simulink model "IdleSpeedSim"  (R2022a)
settings: Solver=FixedStepAuto  StartTime=0.0  StopTime=80  FixedStep=0.01  RelTol=1e-2  EnableMultiTasking=on
InitFcn:
  | IdleSpeedSimParameters
StopFcn:
  | IdleSpeedAutoGrading
values from neighbouring files (symbols this model uses):
  Cd = 0.5    [IdleSpeedSimParameters.m]
  gamma = 1.4    [IdleSpeedSimParameters.m]
  Hu = 42800    [IdleSpeedSimParameters.m]
  J = 1    [IdleSpeedSimParameters.m]
  pambient = 1.013e5    (= 101300)    [IdleSpeedSimParameters.m]
  R = 287e-3    (= 0.287)    [IdleSpeedSimParameters.m]    (also in LQR_Gains.m = [11.13e4 0;0 1])
  T = 294    [IdleSpeedSimParameters.m]
  Vd = 4.6e-3    (= 0.0046)    [IdleSpeedSimParameters.m]
  Vi = 7.36e-3    (= 0.00736)    [IdleSpeedSimParameters.m]
libraries: simulink x1
settings Model: Creator=burl  LastModifiedBy=prajw
settings SolverCC: AlgebraicLoopSolver=TrustRegion
settings DataIOCC: LimitDataPoints=on  SaveFormat=Array  ReturnWorkspaceOutputs=off
settings OptimizationCC: BlockReduction=off  OptimizeBlockIOStorage=off  BufferReuse=off  GlobalBufferReuse=off  ExpressionFolding=off  LocalBlockOutputs=off  LifeSpan=inf  OptimizeDataStoreBuffers=off  BusAssignmentInplaceUpdate=off
settings DebuggingCC: UnderspecifiedInitializationDetection=Classic  MergeDetectMultiDrivingBlocksExec=none  SolverPrmCheckMsg=warning  UnconnectedInputMsg=warning  UnconnectedOutputMsg=warning  UnconnectedLineMsg=warning  StateNameClashWarn=warning  PregeneratedLibrarySubsystemCodeDiagnostic=none  SFUnexpectedBacktrackingDiag=warning  SFNoUnconditionalDefaultTransitionDiag=warning  SFExecutionAtInitializationDiag=none  SFMachineParentedDataDiag=warning  ArithmeticOperatorsInVariantConditions=warning
settings HardwareCC: ProdBitPerPointer=32  ProdBitPerSizeT=32  ProdBitPerPtrDiffT=32  ProdLargestAtomicFloat=None  ProdWordSize=32  ProdHWDeviceType=Generic->Custom  TargetIntDivRoundTo=Zero  TargetEndianess=LittleEndian  TargetHWDeviceType=Generic->Custom
settings ModelReferenceCC: PropagateSignalLabelsOutOfModel=off
settings SFSimCC: SimUseLocalCustomCode=off  CustomCodeUndefinedFunction=UseInterfaceOnly
settings RTWCC: Description=dSPACE DS1006 Hardware Platform  SystemTargetFile=rti1006.tlc  MakeCommand=make_rti  TemplateMakefile=rti1006.tmf  RTWUseLocalCustomCode=off
settings CodeAppCC: StateflowObjectComments=on
settings STFCustomTargetCC: ParMdlRefBuildCompliant=on  MatFileLogging=on  CPPClassGenCompliant=on  SystemTargetFile=rti1006.tlc
settings GRTTargetCC: TargetLangStandard=C89/C90 (ANSI)  CompOptLevelCompliant=off  ConcurrentExecutionCompliant=off  CombineOutputUpdateFcns=off  GRTInterface=on  UseToolchainInfoCompliant=off
settings ConfigComp: CovMetricSettings=dw  CovSaveCumulativeToWorkspaceVar=on  CovSaveSingleToWorkspaceVar=on  CovExternalEMLEnable=off

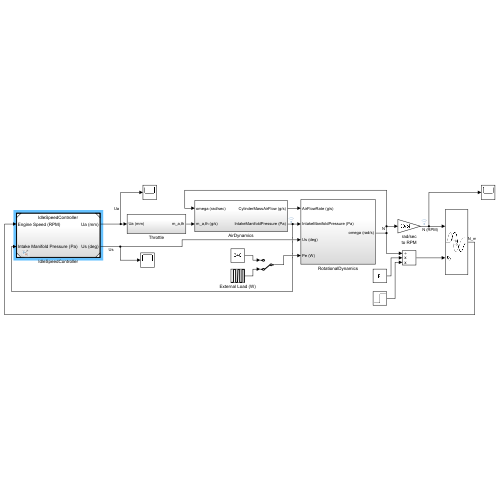
[thumbnail: Simulink's stored preview of the top-level diagram]
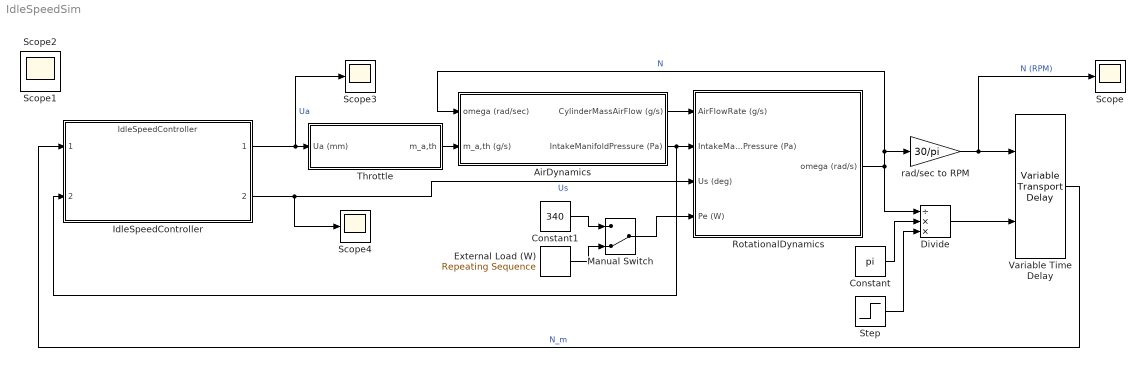
== system IdleSpeedSim ==
  AirDynamics : Subsystem
  Constant : Constant  Value=pi
  Constant1 : Constant  Value=340
  Divide : Product  Inputs=/**
  External Load (W) : simulink/Sources/Repeating Sequence  rep_seq_t=[0 20 20.1 40 40.1]  rep_seq_y=[340 340 1940 1940 340]
  IdleSpeedController : ModelReference  ModelNameDialog=IdleSpeedController  SimulationMode=Normal  ModelReferenceVersion=7.4
  Manual Switch : ManualSwitch  CurrentSetting=0
  RotationalDynamics : Subsystem
  Scope{,1..4} (5 alike) : Scope
  Step : Step  SampleTime=0
  Throttle : Subsystem
  Variable Time Delay : VariableTransportDelay  MaximumDelay=10  ZeroDelay=on
  rad/sec to RPM : Gain  Gain=30/pi
  wires:
  RotationalDynamics/1(omega (rad/s)) -> Divide/1, AirDynamics/1(omega (rad/sec)), rad/sec to RPM/1  "N"
  Variable Time Delay/1 -> IdleSpeedController/1  "N_m"
  IdleSpeedController/1 -> Scope3/1, Throttle/1(Ua (mm))  "Ua"
  Throttle/1(m_a,th) -> AirDynamics/2(m_a,th (g/s))
  AirDynamics/1(CylinderMassAirFlow (g/s)) -> RotationalDynamics/1(AirFlowRate (g/s))
  AirDynamics/2(IntakeManifoldPressure (Pa)) -> IdleSpeedController/2, RotationalDynamics/2(IntakeManifoldPressure (Pa))
  IdleSpeedController/2 -> Scope4/1, RotationalDynamics/3(Us (deg))  "Us"
  Divide/1 -> Variable Time Delay/2
  Constant/1 -> Divide/2
  rad/sec to RPM/1 -> Scope/1, Variable Time Delay/1  "N (RPM)"
  Step/1 -> Divide/3
  Constant1/1 -> Manual Switch/1
  External Load (W)/1 -> Manual Switch/2
  Manual Switch/1 -> RotationalDynamics/4(Pe (W))

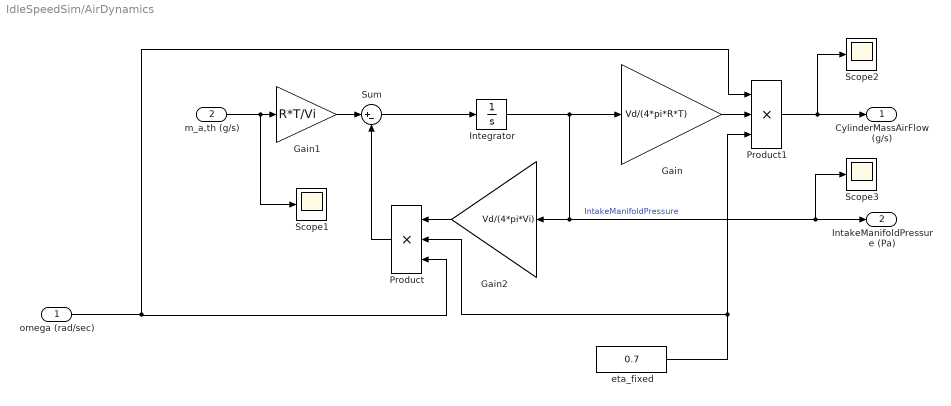
== system IdleSpeedSim/AirDynamics ==
  omega (rad/sec) : Inport
  m_a,th (g/s) : Inport  Port=2
  Gain : Gain  Gain=Vd/(4*pi*R*T)
  Gain1 : Gain  Gain=R*T/Vi
  Gain2 : Gain  Gain=Vd/(4*pi*Vi)
  Integrator : Integrator  InitialCondition=38500
  Product : Product  Inputs=3
  Product1 : Product  Inputs=3
  Scope1 : Scope
  Scope2 : Scope
  Scope3 : Scope
  Sum : Sum  Inputs=|+-
  eta_fixed : Constant  Value=0.7
  CylinderMassAirFlow (g/s) : Outport  VectorParamsAs1DForOutWhenUnconnected=off
  IntakeManifoldPressure (Pa) : Outport  Port=2  VectorParamsAs1DForOutWhenUnconnected=off
  wires:
  m_a,th (g/s)/1 -> Scope1/1, Gain1/1
  Integrator/1 -> Scope3/1, IntakeManifoldPressure (Pa)/1, Gain2/1, Gain/1  "IntakeManifoldPressure"
  Gain1/1 -> Sum/1
  Sum/1 -> Integrator/1
  Gain/1 -> Product1/2
  Product1/1 -> Scope2/1, CylinderMassAirFlow (g/s)/1
  Gain2/1 -> Product/1
  Product/1 -> Sum/2
  eta_fixed/1 -> Product1/3, Product/2
  omega (rad/sec)/1 -> Product1/1, Product/3

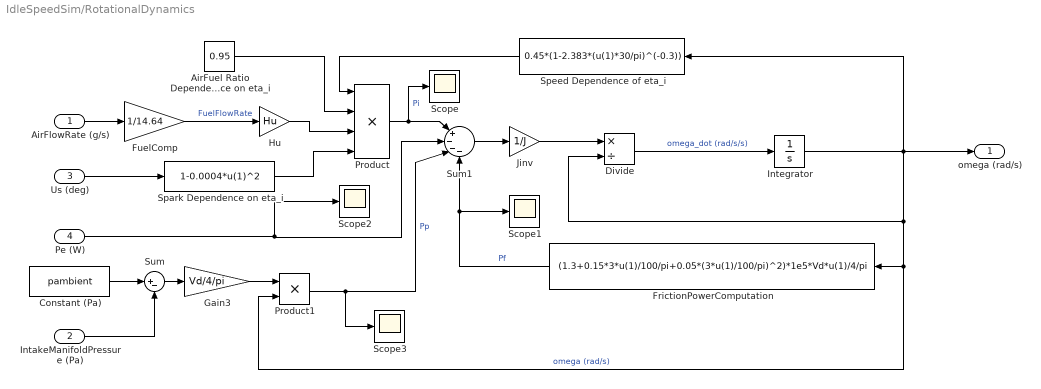
== system IdleSpeedSim/RotationalDynamics ==
  AirFlowRate (g/s) : Inport
  IntakeManifoldPressure (Pa) : Inport  Port=2
  Us (deg) : Inport  Port=3
  Pe (W) : Inport  Port=4
  AirFuel Ratio Dependence on eta_i : Constant  Value=0.95
  Constant (Pa) : Constant  Value=pambient
  Divide : Product  Inputs=*/
  FrictionPowerComputation : Fcn  Expr=(1.3+0.15*3*u(1)/100/pi+0.05*(3*u(1)/100/pi)^2)*1e5*Vd*u(1)/4/pi
  FuelComp : Gain  Gain=1/14.64
  Gain3 : Gain  Gain=Vd/4/pi
  Hu : Gain  Gain=Hu
  Integrator : Integrator  InitialCondition=600*pi/30
  Jinv : Gain  Gain=1/J
  Product : Product  Inputs=4
  Product1 : Product
  Scope{,1..3} (4 alike) : Scope
  Spark Dependence on eta_i : Fcn  Expr=1-0.0004*u(1)^2
  Speed Dependence of eta_i : Fcn  Expr=0.45*(1-2.383*(u(1)*30/pi)^(-0.3))
  Sum : Sum  Inputs=|+-
  Sum1 : Sum  Inputs=|+---
  omega (rad/s) : Outport  VectorParamsAs1DForOutWhenUnconnected=off
  wires:
  Constant (Pa)/1 -> Sum/1
  IntakeManifoldPressure (Pa)/1 -> Sum/2
  Sum/1 -> Gain3/1
  Product1/1 -> Scope3/1, Sum1/3  "Pp"
  AirFlowRate (g/s)/1 -> FuelComp/1
  FuelComp/1 -> Hu/1  "FuelFlowRate"
  Spark Dependence on eta_i/1 -> Product/4
  Hu/1 -> Product/3
  Speed Dependence of eta_i/1 -> Product/1
  Product/1 -> Scope/1, Sum1/1  "Pi"
  Sum1/1 -> Jinv/1
  Us (deg)/1 -> Spark Dependence on eta_i/1
  Integrator/1 -> Divide/2, Product1/2, FrictionPowerComputation/1, omega (rad/s)/1, Speed Dependence of eta_i/1  "omega (rad/s)"
  Gain3/1 -> Product1/1
  FrictionPowerComputation/1 -> Scope1/1, Sum1/4  "Pf"
  Pe (W)/1 -> Sum1/2, Scope2/1
  AirFuel Ratio Dependence on eta_i/1 -> Product/2
  Jinv/1 -> Divide/1
  Divide/1 -> Integrator/1  "omega_dot (rad/s/s)"

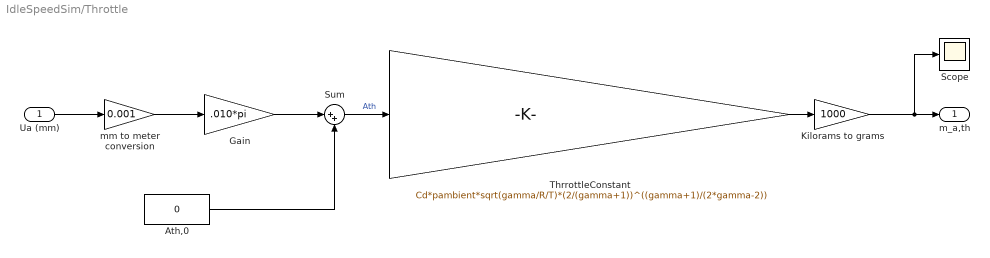
== system IdleSpeedSim/Throttle ==
  Ua (mm) : Inport
  Ath,0 : Constant  Value=0
  Gain : Gain  Gain=.010*pi
  Kilorams to grams : Gain  Gain=1000
  Scope : Scope
  Sum : Sum  Inputs=|++
  ThrrottleConstant : Gain  Gain=Cd*pambient*sqrt(gamma/R/T)*(2/(gamma+1))^((gamma+1)/(2*gamma-2))
  mm to meter conversion : Gain  Gain=0.001
  m_a,th : Outport  VectorParamsAs1DForOutWhenUnconnected=off
  wires:
  Ua (mm)/1 -> mm to meter conversion/1
  Gain/1 -> Sum/1
  Sum/1 -> ThrrottleConstant/1  "Ath"
  Ath,0/1 -> Sum/2
  mm to meter conversion/1 -> Gain/1
  ThrrottleConstant/1 -> Kilorams to grams/1
  Kilorams to grams/1 -> m_a,th/1, Scope/1
